simulink model "amplitude_dependent_delay"  (R2023b)
settings: Solver=VariableStepAuto  StartTime=0.0  StopTime=100.0  MaxStep=0.01  RelTol=1e-6
settings Model: Creator=tom  LastModifiedBy=tom

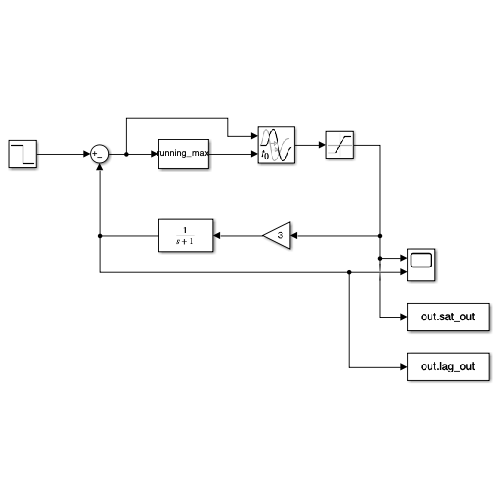
[thumbnail: Simulink's stored preview of the top-level diagram]
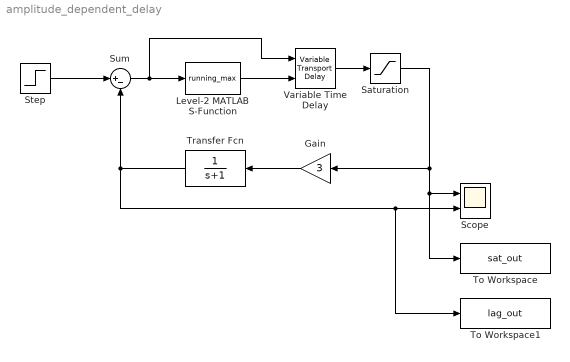
== system amplitude_dependent_delay ==
  Gain : Gain  Gain=3
  Level-2 MATLAB S-Function : M-S-Function  FunctionName=running_max  Parameters=0
  Saturation : Saturate  UpperLimit=1  LowerLimit=-1
  Scope : Scope  NumInputPorts=2
  Step : Step  Before=1  After=0  SampleTime=0
  Sum : Sum  Inputs=|+-
  To Workspace : ToWorkspace  VariableName=sat_out  SampleTime=-1
  To Workspace1 : ToWorkspace  VariableName=lag_out  SampleTime=-1
  Transfer Fcn : TransferFcn  Denominator=[1 1]
  Variable Time Delay : VariableTransportDelay  MaximumDelay=20  ZeroDelay=on
  wires:
  Level-2 MATLAB S-Function/1 -> Variable Time Delay/2
  Sum/1 -> Variable Time Delay/1, Level-2 MATLAB S-Function/1
  Transfer Fcn/1 -> To Workspace1/1, Scope/2, Sum/2
  Step/1 -> Sum/1
  Variable Time Delay/1 -> Saturation/1
  Saturation/1 -> To Workspace/1, Scope/1, Gain/1
  Gain/1 -> Transfer Fcn/1
